simulink model "Hypotenuse_subsystem"  (R2018a)
settings: Solver=VariableStepAuto  StartTime=0.0  StopTime=10.0  RelTol=1e-3
settings Model: Creator=josea  LastModifiedBy=josea

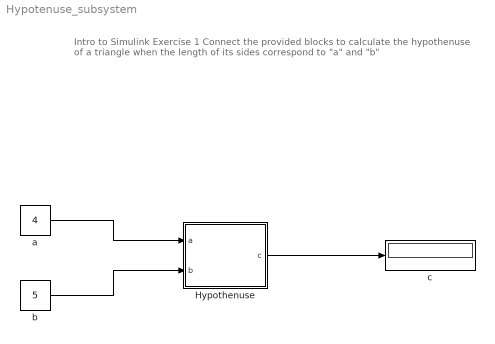
== system Hypotenuse_subsystem ==
  note: Intro to Simulink Exercise 1
      |
      | Connect the provided blocks to calculate the hypothenuse of a triangle when the length of its sides correspond to "a" and "b"
  Hypothenuse : Subsystem
  a : Constant  Value=4
  b : Constant  Value=5
  c : Display
  wires:
  a/1 -> Hypothenuse/1(a)
  b/1 -> Hypothenuse/2(b)
  Hypothenuse/1(c) -> c/1

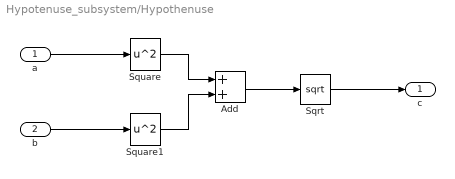
== system Hypotenuse_subsystem/Hypothenuse ==
  a : Inport
  b : Inport  Port=2
  Add : Sum
  Sqrt : Sqrt  SaturateOnIntegerOverflow=on
  Square : Math  Operator=square  SaturateOnIntegerOverflow=on
  Square1 : Math  Operator=square  SaturateOnIntegerOverflow=on
  c : Outport
  wires:
  Sqrt/1 -> c/1
  b/1 -> Square1/1
  Add/1 -> Sqrt/1
  Square1/1 -> Add/2
  Square/1 -> Add/1
  a/1 -> Square/1
